simulink model "mpc_offsets"  (Simulink 6.0)
settings: Solver=ode23s  SolverMode=SingleTasking  StartTime=0.0  StopTime=Tstop  RelTol=1e-3
values from neighbouring files (symbols this model uses):
  x0 = zeros(4,1)    [afti16.m]    (also in misoss.m = [0 0 0 0 0]'; mpcrtwdemo.m = [0 0]')
undefined symbols (not defined in the file or in its folder): r0
libraries: mpclib x1
settings Model: Creator=jowen  LastModifiedBy=jowen  ExtModeTrigMode=oneshot  ExtModeArmWhenConnect=off
settings DataIOCC: LimitDataPoints=off  SignalLoggingName=sigsOut
settings OptimizationCC: BooleanDataType=off
settings DebuggingCC: CheckExecutionContextPreStartOutputMsg=on  CheckExecutionContextRuntimeOutputMsg=on  SolverPrmCheckMsg=none  IntegerOverflowMsg=none
settings HardwareCC: TargetUnknown=on
settings SFSimCC: SFSimApplyToAllLibs=on  SFSimBuildMode=Incremental

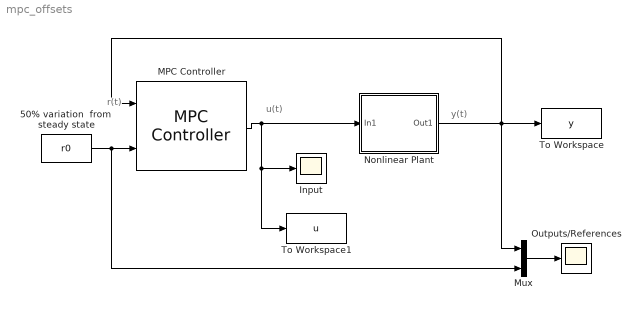
== system mpc_offsets ==
  note: u(t)
  note: y(t)
  note: r(t)
  50% variation  from  steady state : Constant  Value=r0
  Input : Scope
      settings: TimeRange=10  YMin=-8  YMax=2  DataFormat=Structure
  MPC Controller : mpclib/MPC Controller  mpcobj=mpc_controller  n_mv=0  x0=[]  ref_from_ws=off  ref_signal_name=[]  ref_preview=on  md_from_ws=off  md_signal_name=[]  md_preview=on  from_project=off  md_inport=off  project_file=MPCtask.mat
  Mux : Mux  Inputs=2
  Nonlinear Plant : Subsystem  PropExecContextAcrossSSBoundary=on
  Outputs/References : Scope
      settings: TimeRange=10  YMin=-3  YMax=-1.5  DataFormat=Structure
  To Workspace : ToWorkspace  VariableName=y  SampleTime=-1  SaveFormat=Structure With Time
      settings: MaxDataPoints=Inf
  To Workspace1 : ToWorkspace  VariableName=u  SampleTime=-1  SaveFormat=Structure With Time
      settings: MaxDataPoints=Inf
  wires:
  MPC Controller/1 -> Input/1, To Workspace1/1, Nonlinear Plant/1(In1)
  Mux/1 -> Outputs/References/1
  50% variation  from  steady state/1 -> Mux/2, MPC Controller/2
  Nonlinear Plant/1(Out1) -> To Workspace/1, Mux/1, MPC Controller/1

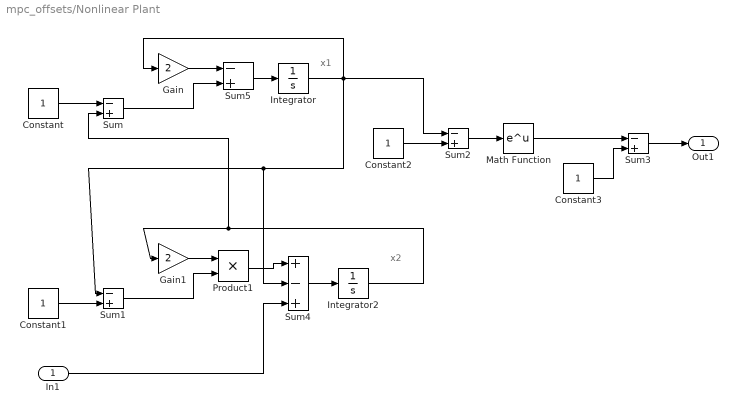
== system mpc_offsets/Nonlinear Plant ==
  note: x1
  note: x2
  In1 : Inport  LatchInput=off
  Constant{,1..3} (4 alike) : Constant
  Gain : Gain  Gain=2  SaturateOnIntegerOverflow=on
  Gain1 : Gain  Gain=2  SaturateOnIntegerOverflow=on
  Integrator : Integrator  InitialCondition=x0(1)  UpperSaturationLimit=Inf  LowerSaturationLimit=-Inf
  Integrator2 : Integrator  InitialCondition=x0(2)  UpperSaturationLimit=Inf  LowerSaturationLimit=-Inf
  Math Function : Math  SaturateOnIntegerOverflow=on
  Product1 : Product  SaturateOnIntegerOverflow=on  InputSameDT=on
  Sum{,1..3,5} (5 alike) : Sum  Inputs=-+  SaturateOnIntegerOverflow=on  InputSameDT=on
  Sum4 : Sum  Inputs=+-+  SaturateOnIntegerOverflow=on  InputSameDT=on
  Out1 : Outport
  wires:
  Sum5/1 -> Integrator/1
  Gain/1 -> Sum5/1
  Integrator/1 -> Gain/1, Sum2/1, Sum1/1, Sum4/2
  Constant/1 -> Sum/1
  Sum/1 -> Sum5/2
  Gain1/1 -> Product1/1
  Sum1/1 -> Product1/2
  Constant1/1 -> Sum1/2
  Constant2/1 -> Sum2/2
  Sum2/1 -> Math Function/1
  Constant3/1 -> Sum3/2
  Math Function/1 -> Sum3/1
  Sum3/1 -> Out1/1
  Integrator2/1 -> Gain1/1, Sum/2
  Sum4/1 -> Integrator2/1
  Product1/1 -> Sum4/1
  In1/1 -> Sum4/3
